simulink model "WindFarm_2023_BaseModel_v2"  (R2019a)
(part 4 of 86)

  BusC6/RConn1 -- Three-Phase Breaker 27/LConn1 -- Three-Phase Breaker 30/LConn1 -- Three-Phase Breaker 55/LConn1 -- Three-Phase Breaker 37/LConn1 -- Three-Phase Breaker 36/LConn1 -- Three-Phase Breaker 34/LConn1 -- Three-Phase Breaker 33/LConn1 -- Three-Phase Breaker 32/LConn1 -- Three-Phase Breaker 31/LConn1
  Three-Phase Breaker 32/LConn2 -- Three-Phase Breaker 31/LConn2 -- Three-Phase Breaker 30/LConn2 -- Three-Phase Breaker 27/LConn2 -- BusC6/RConn2 -- Three-Phase Breaker 33/LConn2 -- Three-Phase Breaker 55/LConn2 -- Three-Phase Breaker 37/LConn2 -- Three-Phase Breaker 36/LConn2 -- Three-Phase Breaker 34/LConn2
  Three-Phase Breaker 39/LConn3 -- BusC10/RConn3 -- Three-Phase Breaker 26/LConn3
  Three-Phase Breaker 40/LConn1 -- Three-Phase Breaker 24/LConn1 -- BusC5/RConn1 -- Three-Phase Breaker 35/LConn1 -- Three-Phase Breaker 45/LConn1 -- Three-Phase Breaker 44/LConn1 -- Three-Phase Breaker 43/LConn1 -- Three-Phase Breaker 42/LConn1 -- Three-Phase Breaker 41/LConn1
  Three-Phase Breaker 41/LConn2 -- Three-Phase Breaker 45/LConn2 -- Three-Phase Breaker 44/LConn2 -- Three-Phase Breaker 43/LConn2 -- Three-Phase Breaker 42/LConn2 -- BusC5/RConn2 -- Three-Phase Breaker 24/LConn2 -- Three-Phase Breaker 35/LConn2 -- Three-Phase Breaker 40/LConn2
  BusC6/LConn3 -- Three-Phase Breaker 28/RConn3 -- Three-Phase Breaker 38/RConn3
  BusC5/LConn2 -- Three-Phase Breaker 25/RConn2 -- Three-Phase Breaker 38/LConn2
  Three-Phase Breaker 28/RConn1 -- BusC6/LConn1 -- Three-Phase Breaker 38/RConn1
  Three-Phase Breaker 35/LConn3 -- BusC5/RConn3 -- Three-Phase Breaker 43/LConn3 -- Three-Phase Breaker 45/LConn3 -- Three-Phase Breaker 44/LConn3 -- Three-Phase Breaker 42/LConn3 -- Three-Phase Breaker 41/LConn3 -- Three-Phase Breaker 40/LConn3 -- Three-Phase Breaker 24/LConn3
  Three-Phase Breaker 39/LConn2 -- BusC10/RConn2 -- Three-Phase Breaker 26/LConn2
  Three-Phase Breaker 28/RConn2 -- Three-Phase Breaker 38/RConn2 -- BusC6/LConn2
  BusC5/LConn3 -- Three-Phase Breaker 25/RConn3 -- Three-Phase Breaker 38/LConn3
  BusC5/LConn1 -- Three-Phase Breaker 25/RConn1 -- Three-Phase Breaker 38/LConn1
  Three-Phase Breaker 39/LConn1 -- Three-Phase Breaker 26/LConn1 -- BusC10/RConn1
  5 km series28/LConn2 -- Three-Phase Breaker 27/RConn2
  Three-Phase Breaker 26/RConn2 -- " 5"/LConn2
  Three-Phase Breaker 39/RConn2 -- BusC11/LConn2 -- Three-Phase Breaker 29/LConn2
  5 km series29/RConn3 -- Wind Type IV Detailed v2.1 - 27/LConn3
  5 km series29/RConn2 -- Wind Type IV Detailed v2.1 - 27/LConn2
  5 km series33/LConn1 -- Three-Phase Breaker 24/RConn1
  Three-Phase Breaker 29/RConn1 -- " 6"/LConn1
  5 km series29/LConn2 -- Three-Phase Breaker 32/RConn2
  5 km series28/RConn3 -- Wind Type IV Detailed v2.1 - 24/LConn3
  Three-Phase Breaker 28/LConn1 -- " 6"/RConn1
  5 km series25/LConn2 -- Three-Phase Breaker 37/RConn2
  5 km series26/LConn3 -- Three-Phase Breaker 36/RConn3
  Three-Phase Breaker 28/LConn3 -- " 6"/RConn3
  5 km series25/LConn1 -- Three-Phase Breaker 37/RConn1
  5 km series25/RConn2 -- Wind Type IV Detailed v2.1 - 23/LConn2
  5 km series29/LConn3 -- Three-Phase Breaker 32/RConn3
  5 km series35/RConn2 -- Wind Type IV Detailed v2.1 - 32/LConn2
  Three-Phase Breaker 28/LConn2 -- " 6"/RConn2
  5 km series24/RConn1 -- Wind Type IV Detailed v2.1 - 28/LConn1
  5 km series27/RConn1 -- Wind Type IV Detailed v2.1 - 25/LConn1
  5 km series29/RConn1 -- Wind Type IV Detailed v2.1 - 27/LConn1
  5 km series29/LConn1 -- Three-Phase Breaker 32/RConn1
  Three-Phase Breaker 39/RConn1 -- BusC11/LConn1 -- Three-Phase Breaker 29/LConn1
  5 km series27/LConn3 -- Three-Phase Breaker 30/RConn3
  5 km series32/RConn3 -- Wind Type IV Detailed v2.1 - 31/LConn3
  5 km series27/LConn2 -- Three-Phase Breaker 30/RConn2
  5 km series24/LConn3 -- Three-Phase Breaker 33/RConn3
  5 km series24/RConn2 -- Wind Type IV Detailed v2.1 - 28/LConn2
  5 km series26/RConn1 -- Wind Type IV Detailed v2.1 - 22/LConn1
  5 km series25/RConn3 -- Wind Type IV Detailed v2.1 - 23/LConn3
  5 km series24/RConn3 -- Wind Type IV Detailed v2.1 - 28/LConn3
  5 km series30/RConn1 -- Wind Type IV Detailed v2.1 - 26/LConn1
  5 km series25/LConn3 -- Three-Phase Breaker 37/RConn3
  5 km series26/RConn3 -- Wind Type IV Detailed v2.1 - 22/LConn3
  5 km series30/LConn2 -- Three-Phase Breaker 31/RConn2
  5 km series35/LConn3 -- Three-Phase Breaker 40/RConn3
  5 km series31/RConn3 -- Wind Type IV Detailed v2.1 - 29/LConn3
  5 km series28/RConn1 -- Wind Type IV Detailed v2.1 - 24/LConn1
  5 km series35/RConn3 -- Wind Type IV Detailed v2.1 - 32/LConn3
  5 km series28/RConn2 -- Wind Type IV Detailed v2.1 - 24/LConn2
  5 km series27/LConn1 -- Three-Phase Breaker 30/RConn1
  5 km series31/LConn1 -- Three-Phase Breaker 34/RConn1
  5 km series22/LConn3 -- Three-Phase Breaker 45/RConn3
  5 km series32/RConn1 -- Wind Type IV Detailed v2.1 - 31/LConn1
  5 km series30/LConn1 -- Three-Phase Breaker 31/RConn1
  5 km series26/LConn2 -- Three-Phase Breaker 36/RConn2
  5 km series33/RConn1 -- Wind Type IV Detailed v2.1 - 30/LConn1
  5 km series31/RConn2 -- Wind Type IV Detailed v2.1 - 29/LConn2
  5 km series32/LConn1 -- Three-Phase Breaker 35/RConn1
  5 km series23/LConn3 -- Three-Phase Breaker 44/RConn3
  Three-Phase Breaker 39/RConn3 -- Three-Phase Breaker 29/LConn3 -- BusC11/LConn3
  5 km series26/RConn2 -- Wind Type IV Detailed v2.1 - 22/LConn2
  5 km series21/LConn2 -- Three-Phase Breaker 42/RConn2
  5 km series21/LConn1 -- Three-Phase Breaker 42/RConn1
  5 km series23/LConn1 -- Three-Phase Breaker 44/RConn1
  5 km series31/LConn3 -- Three-Phase Breaker 34/RConn3
  5 km series22/LConn1 -- Three-Phase Breaker 45/RConn1
  5 km series33/RConn2 -- Wind Type IV Detailed v2.1 - 30/LConn2
  5 km series36/RConn3 -- Wind Type IV Detailed v2.1 - 35/LConn3
  5 km series24/LConn1 -- Three-Phase Breaker 33/RConn1
  Three-Phase Breaker 29/RConn2 -- " 6"/LConn2
  5 km series22/RConn2 -- Wind Type IV Detailed v2.1 - 21/LConn2
  5 km series35/RConn1 -- Wind Type IV Detailed v2.1 - 32/LConn1
  5 km series36/LConn2 -- Three-Phase Breaker 43/RConn2
  5 km series34/RConn2 -- Wind Type IV Detailed v2.1 - 33/LConn2
  5 km series36/LConn1 -- Three-Phase Breaker 43/RConn1
  5 km series34/RConn1 -- Wind Type IV Detailed v2.1 - 33/LConn1
  5 km series28/LConn1 -- Three-Phase Breaker 27/RConn1
  5 km series35/LConn1 -- Three-Phase Breaker 40/RConn1
  5 km series27/RConn2 -- Wind Type IV Detailed v2.1 - 25/LConn2
  5 km series23/RConn2 -- Wind Type IV Detailed v2.1 - 20/LConn2
  5 km series36/RConn2 -- Wind Type IV Detailed v2.1 - 35/LConn2
  Three-Phase Breaker 25/LConn2 -- " 5"/RConn2
  Three-Phase Breaker 29/RConn3 -- " 6"/LConn3
  5 km series24/LConn2 -- Three-Phase Breaker 33/RConn2
  5 km series36/RConn1 -- Wind Type IV Detailed v2.1 - 35/LConn1
  5 km series34/RConn3 -- Wind Type IV Detailed v2.1 - 33/LConn3
  5 km series34/LConn1 -- Three-Phase Breaker 41/RConn1
  5 km series32/LConn3 -- Three-Phase Breaker 35/RConn3
  5 km series28/LConn3 -- Three-Phase Breaker 27/RConn3
  Three-Phase Breaker 26/RConn3 -- " 5"/LConn3
  Three-Phase Breaker 26/RConn1 -- " 5"/LConn1
  5 km series33/RConn3 -- Wind Type IV Detailed v2.1 - 30/LConn3
  5 km series33/LConn3 -- Three-Phase Breaker 24/RConn3
  5 km series30/RConn3 -- Wind Type IV Detailed v2.1 - 26/LConn3
  Three-Phase Breaker 25/LConn3 -- " 5"/RConn3
  5 km series27/RConn3 -- Wind Type IV Detailed v2.1 - 25/LConn3
  5 km series34/LConn3 -- Three-Phase Breaker 41/RConn3
  5 km series22/RConn3 -- Wind Type IV Detailed v2.1 - 21/LConn3
  5 km series23/LConn2 -- Three-Phase Breaker 44/RConn2
  5 km series22/LConn2 -- Three-Phase Breaker 45/RConn2
  5 km series21/RConn2 -- Wind Type IV Detailed v2.1 - 34/LConn2
  5 km series21/LConn3 -- Three-Phase Breaker 42/RConn3
  Three-Phase Breaker 25/LConn1 -- " 5"/RConn1
  5 km series31/RConn1 -- Wind Type IV Detailed v2.1 - 29/LConn1
  5 km series33/LConn2 -- Three-Phase Breaker 24/RConn2
  5 km series30/LConn3 -- Three-Phase Breaker 31/RConn3
  5 km series32/RConn2 -- Wind Type IV Detailed v2.1 - 31/LConn2
  5 km series21/RConn3 -- Wind Type IV Detailed v2.1 - 34/LConn3
  5 km series32/LConn2 -- Three-Phase Breaker 35/RConn2
  5 km series21/RConn1 -- Wind Type IV Detailed v2.1 - 34/LConn1
  5 km series25/RConn1 -- Wind Type IV Detailed v2.1 - 23/LConn1
  5 km series23/RConn1 -- Wind Type IV Detailed v2.1 - 20/LConn1
  5 km series23/RConn3 -- Wind Type IV Detailed v2.1 - 20/LConn3
  5 km series31/LConn2 -- Three-Phase Breaker 34/RConn2
  5 km series26/LConn1 -- Three-Phase Breaker 36/RConn1
  5 km series35/LConn2 -- Three-Phase Breaker 40/RConn2
  5 km series36/LConn3 -- Three-Phase Breaker 43/RConn3
  5 km series30/RConn2 -- Wind Type IV Detailed v2.1 - 26/LConn2
  5 km series22/RConn1 -- Wind Type IV Detailed v2.1 - 21/LConn1
  5 km series34/LConn2 -- Three-Phase Breaker 41/RConn2
  Three-Phase Breaker 23/LConn2 -- BusC8/RConn2 -- Three-Phase Breaker 11/LConn2
  Three-Phase Breaker 23/LConn1 -- BusC8/RConn1 -- Three-Phase Breaker 11/LConn1
  Three-Phase Breaker 49/RConn1 -- BusC8/LConn1
  Three-Phase Breaker 49/RConn2 -- BusC8/LConn2
  Three-Phase Breaker 49/RConn3 -- BusC8/LConn3
  BusC11/RConn3 -- Three-Phase Breaker 46/RConn3
  BusC11/RConn2 -- Three-Phase Breaker 46/RConn2
  Three-Phase Breaker 48/RConn1 -- BusC10/LConn1
  Three-Phase Breaker 48/RConn2 -- BusC10/LConn2
  Three-Phase Breaker 48/RConn3 -- BusC10/LConn3
  Three-Phase Breaker 46/RConn1 -- BusC11/RConn1
  Three-Phase Breaker 47/LConn1 -- 5 km series38/RConn1
  Three-Phase Breaker 47/LConn2 -- 5 km series38/RConn2
  5 km series38/RConn3 -- Three-Phase Breaker 47/LConn3
  Three-Phase Breaker 48/LConn1 -- 5 km series39/RConn1
  5 km series39/RConn2 -- Three-Phase Breaker 48/LConn2
  5 km series39/RConn3 -- Three-Phase Breaker 48/LConn3
  Three-Phase Breaker 46/LConn1 -- 5 km series40/RConn1
  Three-Phase Breaker 46/LConn2 -- 5 km series40/RConn2
  Three-Phase Breaker 46/LConn3 -- 5 km series40/RConn3
  Three-Phase Breaker 49/LConn1 -- 5 km series37/RConn1
  Three-Phase Breaker 49/LConn2 -- 5 km series37/RConn2
  Three-Phase Breaker 49/LConn3 -- 5 km series37/RConn3
  Three-Phase Breaker 50/RConn1 -- 5 km series37/LConn1
  Three-Phase Breaker 50/RConn2 -- 5 km series37/LConn2
  Three-Phase Breaker 50/RConn3 -- 5 km series37/LConn3
  Three-Phase Breaker 51/RConn1 -- 5 km series38/LConn1
  Three-Phase Breaker 51/RConn2 -- 5 km series38/LConn2
  Three-Phase Breaker 51/RConn3 -- 5 km series38/LConn3
  Three-Phase Breaker 52/RConn1 -- 5 km series39/LConn1
  Three-Phase Breaker 52/RConn2 -- 5 km series39/LConn2
  Three-Phase Breaker 52/RConn3 -- 5 km series39/LConn3
  Three-Phase Breaker 53/RConn1 -- 5 km series40/LConn1
  Three-Phase Breaker 53/RConn2 -- 5 km series40/LConn2
  Three-Phase Breaker 53/RConn3 -- 5 km series40/LConn3
  Three-Phase Breaker 50/LConn1 -- Three-Phase Breaker 51/LConn1 -- Three-Phase Breaker 52/LConn1 -- Three-Phase Breaker 53/LConn1 -- BusC7/RConn1
  Three-Phase Breaker 50/LConn2 -- Three-Phase Breaker 51/LConn2 -- Three-Phase Breaker 52/LConn2 -- Three-Phase Breaker 53/LConn2 -- BusC7/RConn2
  Three-Phase Breaker 50/LConn3 -- Three-Phase Breaker 53/LConn3 -- Three-Phase Breaker 52/LConn3 -- Three-Phase Breaker 51/LConn3 -- BusC7/RConn3
  5 km series41/LConn2 -- Three-Phase Breaker 54/RConn2
  5 km series41/RConn1 -- Wind Type IV Detailed v2.1 - 36/LConn1
  5 km series41/LConn1 -- Three-Phase Breaker 54/RConn1
  5 km series41/LConn3 -- Three-Phase Breaker 54/RConn3
  5 km series41/RConn2 -- Wind Type IV Detailed v2.1 - 36/LConn2
  5 km series41/RConn3 -- Wind Type IV Detailed v2.1 - 36/LConn3
  5 km series42/LConn2 -- Three-Phase Breaker 55/RConn2
  5 km series42/RConn1 -- Wind Type IV Detailed v2.1 - 37/LConn1
  5 km series42/LConn1 -- Three-Phase Breaker 55/RConn1
  5 km series42/LConn3 -- Three-Phase Breaker 55/RConn3
  5 km series42/RConn2 -- Wind Type IV Detailed v2.1 - 37/LConn2
  5 km series42/RConn3 -- Wind Type IV Detailed v2.1 - 37/LConn3
  Three-Phase Breaker 58/RConn3 -- 5 km series3/LConn3
  Three-Phase Breaker 59/RConn3 -- 5 km series4/LConn3
  Three-Phase Breaker 57/LConn1 -- 5 km series3/RConn1
  Three-Phase Breaker 58/RConn2 -- 5 km series3/LConn2
  5 km series4/RConn3 -- Three-Phase Breaker 56/LConn3
  Three-Phase Breaker 58/RConn1 -- 5 km series3/LConn1
  Three-Phase Breaker 59/RConn1 -- 5 km series4/LConn1
  Three-Phase Breaker 57/LConn2 -- 5 km series3/RConn2
  Three-Phase Breaker 56/LConn1 -- 5 km series4/RConn1
  Three-Phase Breaker 57/LConn3 -- 5 km series3/RConn3
  Three-Phase Breaker 56/LConn2 -- 5 km series4/RConn2
  Three-Phase Breaker 59/RConn2 -- 5 km series4/LConn2
  Three-Phase Breaker 58/LConn2 -- Three-Phase Breaker 59/LConn2 -- 2500 MVA X0/X1=2/RConn3
  Three-Phase Breaker 58/LConn3 -- 2500 MVA X0/X1=2/RConn2 -- Three-Phase Breaker 59/LConn3
  Three-Phase Breaker 58/LConn1 -- 2500 MVA X0/X1=2/RConn1 -- Three-Phase Breaker 59/LConn1
  BusC7/LConn1 -- Three-Phase Breaker 56/RConn1 -- Three-Phase Breaker 57/RConn1
  BusC7/LConn2 -- Three-Phase Breaker 56/RConn2 -- Three-Phase Breaker 57/RConn2
  BusC7/LConn3 -- Three-Phase Breaker 56/RConn3 -- Three-Phase Breaker 57/RConn3
